simulink model "reverbcomb"  (Simulink 7.7)
settings: Solver=FixedStepDiscrete  StartTime=0.0  StopTime=10  MaxStep=1/50  RelTol=1e-3
libraries: simulink x2, dspsrcs4 x1, dspmtrx3 x1, dspwin32 x1
settings Model: Creator=jlukito  LastModifiedBy=Arun
settings OptimizationCC: InitFltsAndDblsToZero=on
settings DebuggingCC: SaveWithParameterizedLinksMsg=none  StrictBusMsg=Warning
settings HardwareCC: TargetHWDeviceType=32-bit Generic
settings GRTTargetCC: TargetFcnLib=ansi_tfl_tmw.mat

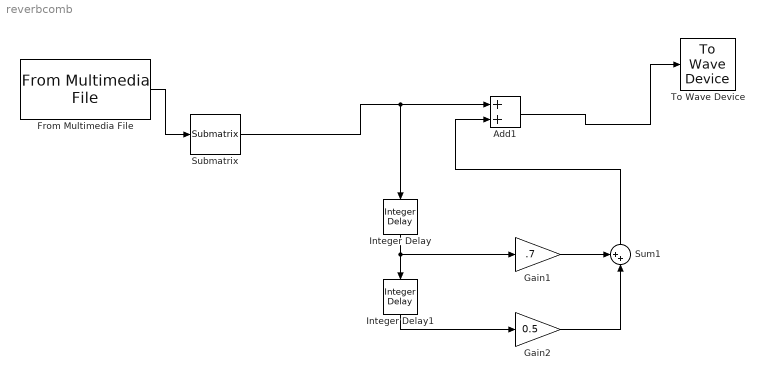
== system reverbcomb ==
  Add1 : Sum
  From Multimedia File : dspsrcs4/From Multimedia File  inputFilename=I:\Documents and Settings\Arun\Desktop\monayi\speech_dft.wav  loop=on  numPlays=1  outputStreams=Audio only  videoDataType=single  audioDataType=double  inheritSampleTime=on  userDefinedSampleTime=1/30  noAudioOutput=off  isIntensityVideo=off  fourcc=RGB  colorVideoFormat=Separate color signals  outputEOF=off  dataOrg=Column-major  audioFrameSize=1  computeAudioFrameSize=off
  Gain1 : Gain  Gain=.7
  Gain2 : Gain  Gain=0.5
  Integer Delay : simulink/Discrete/Integer Delay  NumDelays=700  InputProcessing=Inherited  vinit=0.0  samptime=-1
  Integer Delay1 : simulink/Discrete/Integer Delay  NumDelays=200  InputProcessing=Inherited  vinit=0.0  samptime=-1
  Submatrix : dspmtrx3/Submatrix  RowSpan=All rows  RowStartMode=First  RowStartIndex=1  RowEndMode=Last  RowEndIndex=1  ColSpan=One column  ColStartMode=First  ColStartIndex=1  ColEndMode=Last  ColEndIndex=1
  Sum1 : Sum  Inputs=++|
  To Wave Device : dspwin32/To Wave Device  bufDuration=2  determineBufSize=on  userIntBufSize=256  initDelay=0.1  useDefaultDevice=on  userDeviceID=Microsoft RDP Audio Driver  enable24Bit=off
  wires:
  Integer Delay/1 -> Gain1/1, Integer Delay1/1
  Gain1/1 -> Sum1/1
  Integer Delay1/1 -> Gain2/1
  Gain2/1 -> Sum1/2
  Sum1/1 -> Add1/2
  Add1/1 -> To Wave Device/1
  From Multimedia File/1 -> Submatrix/1
  Submatrix/1 -> Add1/1, Integer Delay/1
